simulink model "tanks3"  (R2025b)
settings: Solver=VariableStepAuto  StartTime=0.0  StopTime=10.0  RelTol=1e-3
model workspace (MAT data in the model file):
  sine_amp = 0.2
settings Model: Creator=jbrouill  LastModifiedBy=seby
settings SolverCC: AlgebraicLoopSolver=TrustRegion
settings DataIOCC: Refine=10
settings DebuggingCC: UnconnectedInputMsg=warning  UnconnectedOutputMsg=warning  UnconnectedLineMsg=warning
settings ModelReferenceCC: EnableRefExpFcnMdlSchedulingChecks=on
settings RTWCC: GPUComputeCapability=3.5

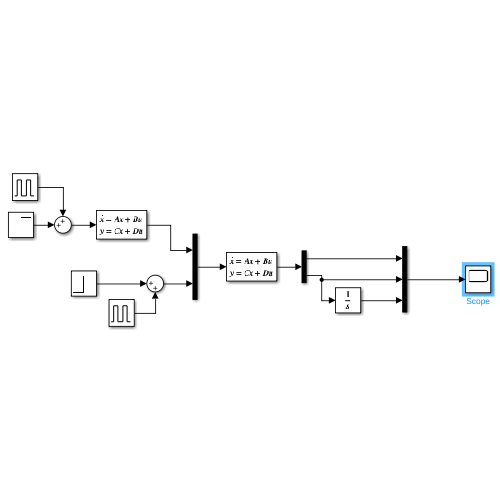
[thumbnail: Simulink's stored preview of the top-level diagram]
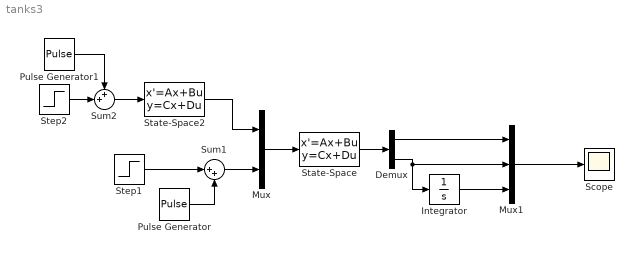
== system tanks3 ==
  Demux : Demux  Outputs=2
  Integrator : Integrator
  Mux : Mux  Inputs=2
  Mux1 : Mux  Inputs=3
  Pulse Generator : DiscretePulseGenerator  PulseType=Time based  Amplitude=0.4  Period=3  PulseWidth=50
  Pulse Generator1 : DiscretePulseGenerator  PulseType=Time based  Amplitude=0.25  PulseWidth=50
  Scope : Scope
      settings: ActiveDisplayYMinimum=-23.172596782396361  ActiveDisplayYMaximum=67.59303695753465
  State-Space : StateSpace  A=[-3 0; 3 -5]  B=[1 0 ; 0 1]  C=[3 0 ; 0 5]  D=zeros(2,2)  InitialCondition=[0.1 ; 0.1]
  State-Space2 : StateSpace  A=-2/3  B=5/3  C=2  D=0  InitialCondition=0.1
  Step1 : Step  Time=0  After=0.5  SampleTime=0
  Step2 : Step  Time=0  After=1.5  SampleTime=0
  Sum1 : Sum  Inputs=|++
  Sum2 : Sum  Inputs=++|
  wires:
  Sum1/1 -> Mux/2
  Step1/1 -> Sum1/1
  Pulse Generator/1 -> Sum1/2
  Mux/1 -> State-Space/1
  State-Space2/1 -> Mux/1
  Sum2/1 -> State-Space2/1
  Pulse Generator1/1 -> Sum2/1
  Step2/1 -> Sum2/2
  State-Space/1 -> Demux/1
  Demux/2 -> Mux1/2, Integrator/1
  Integrator/1 -> Mux1/3
  Mux1/1 -> Scope/1
  Demux/1 -> Mux1/1
